simulink model "DIas"  (R2020a)
settings: Solver=VariableStepAuto  StartTime=0.0  StopTime=1E-4  RelTol=1e-6
InitFcn:
  | R1 = 1000;
  | R2 = 20;
  | L = 25.3E-6;
  | C = 100E-9;
  | IS = 1E-8;
  | UT = 26E-3;
  | f = 0.15E+6;
  | 
  | N = 10;
  | uMax = 3.84E-2;
  | uas = linspace(0, uMax, N);
  | ias = IS * (exp(uas/UT) - 1);
settings Model: Creator=LKP  LastModifiedBy=peter

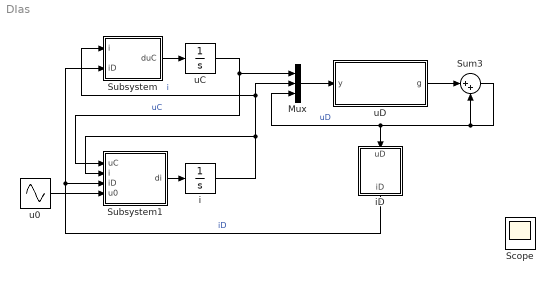
== system DIas ==
  Mux : Mux  Inputs=3
  Subsystem : Subsystem
  Subsystem1 : Subsystem
  Sum3 : Sum  Inputs=|++
  i : Integrator
  iD : Subsystem
      mask Display: disp('iD(uD)')
  u0 : Sin  Amplitude=-1  Frequency=2*pi*f  SampleTime=0
  uC : Integrator
  uD : Subsystem
      mask Display: disp('g(uC, i, uD)')
  Scope : Scope
  wires:
  i/1 -> Mux/2, Subsystem/1(i), Subsystem1/2(i)  "i"
  iD/1(iD) -> Subsystem/2(iD), Subsystem1/3(iD)  "iD"
  uC/1 -> Subsystem1/1(uC), Mux/1  "uC"
  uD/1(g) -> Sum3/1
  Sum3/1 -> Sum3/2, Mux/3, iD/1(uD)  "uD"
  Mux/1 -> uD/1(y)
  Subsystem/1(duC) -> uC/1
  Subsystem1/1(di) -> i/1
  u0/1 -> Subsystem1/4(u0)

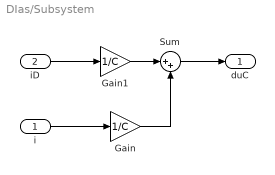
== system DIas/Subsystem ==
  i : Inport
  iD : Inport  Port=2
  Gain : Gain  Gain=1/C
  Gain1 : Gain  Gain=1/C
  Sum : Sum  Inputs=|++
  duC : Outport
  wires:
  i/1 -> Gain/1
  iD/1 -> Gain1/1
  Gain1/1 -> Sum/1
  Gain/1 -> Sum/2
  Sum/1 -> duC/1

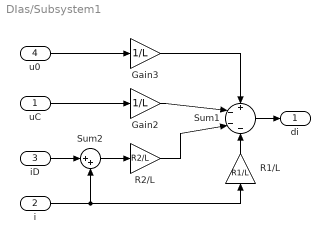
== system DIas/Subsystem1 ==
  uC : Inport
  i : Inport  Port=2
  iD : Inport  Port=3
  u0 : Inport  Port=4
  Gain2 : Gain  Gain=1/L
  Gain3 : Gain  Gain=1/L
  R1/L : Gain  Gain=R1/L
  R2/L : Gain  Gain=R2/L
  Sum1 : Sum  Inputs=+---
  Sum2 : Sum  Inputs=|++
  di : Outport
  wires:
  Gain2/1 -> Sum1/2
  R2/L/1 -> Sum1/3
  uC/1 -> Gain2/1
  Sum2/1 -> R2/L/1
  i/1 -> R1/L/1, Sum2/2
  Gain3/1 -> Sum1/1
  iD/1 -> Sum2/1
  R1/L/1 -> Sum1/4
  u0/1 -> Gain3/1
  Sum1/1 -> di/1

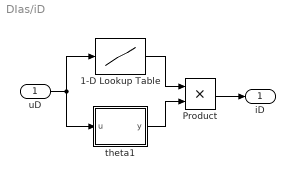
== system DIas/iD ==
  uD : Inport
  1-D Lookup Table : Lookup_n-D  NumberOfTableDimensions=1  BreakpointsForDimension1=uas  Table=IS * (exp(uas/UT) - 1)  InternalRulePriority=Speed  RndMeth=Simplest  InputSameDT=on
  Product : Product
  theta1 : Subsystem
      mask Display: text(0.5,0.5,'\fontsize{20}\Theta', 'texmode', 'on','horizontalAlignment', 'center', 'verticalAlignment', 'middle')
  iD : Outport
  wires:
  uD/1 -> theta1/1(u), 1-D Lookup Table/1
  1-D Lookup Table/1 -> Product/1
  Product/1 -> iD/1
  theta1/1(y) -> Product/2

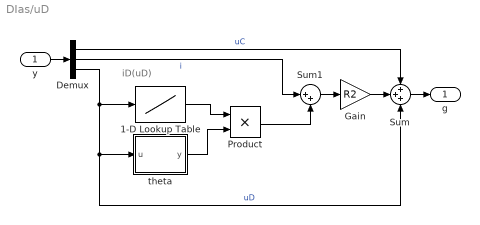
== system DIas/uD ==
  note: iD(uD)
  y : Inport
  1-D Lookup Table : Lookup_n-D  NumberOfTableDimensions=1  BreakpointsForDimension1=uas  Table=IS * (exp(uas/UT) - 1)  InternalRulePriority=Speed  RndMeth=Simplest  InputSameDT=on
  Demux : Demux  Outputs=3
  Gain : Gain  Gain=R2
  Product : Product
  Sum : Sum  Inputs=+++
  Sum1 : Sum  Inputs=|++
  theta : Subsystem
      mask Display: text(0.5,0.5,'\fontsize{20}\Theta', 'texmode', 'on','horizontalAlignment', 'center', 'verticalAlignment', 'middle')
  g : Outport
  wires:
  y/1 -> Demux/1
  Demux/1 -> Sum/1  "uC"
  Gain/1 -> Sum/2
  Demux/2 -> Sum1/1  "i"
  Product/1 -> Sum1/2
  Sum1/1 -> Gain/1
  1-D Lookup Table/1 -> Product/1
  Demux/3 -> 1-D Lookup Table/1, theta/1(u), Sum/3  "uD"
  theta/1(y) -> Product/2
  Sum/1 -> g/1

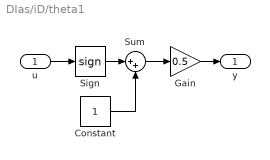
== system DIas/iD/theta1 ==
  u : Inport
  Constant : Constant
  Gain : Gain  Gain=0.5
  Sign : Signum
  Sum : Sum  Inputs=|++
  y : Outport
  wires:
  Sum/1 -> Gain/1
  u/1 -> Sign/1
  Constant/1 -> Sum/2
  Sign/1 -> Sum/1
  Gain/1 -> y/1

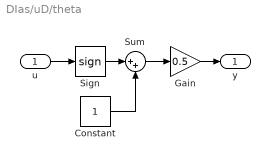
== system DIas/uD/theta ==
  u : Inport
  Constant : Constant
  Gain : Gain  Gain=0.5
  Sign : Signum
  Sum : Sum  Inputs=|++
  y : Outport
  wires:
  Sum/1 -> Gain/1
  u/1 -> Sign/1
  Constant/1 -> Sum/2
  Sign/1 -> Sum/1
  Gain/1 -> y/1
